simulink model "xo_test"  (R2023a)
settings: Solver=VariableStepAuto  StartTime=0.0  StopTime=10.0  RelTol=1e-3
PreLoadFcn:
  | xo = importrobot('urdf/alpha4_LC_FB_XYZ.urdf');
  | xo.DataFormat = 'col';
libraries: robotmaniplib x72, RoboticsCode x72
(part 2 of 2)

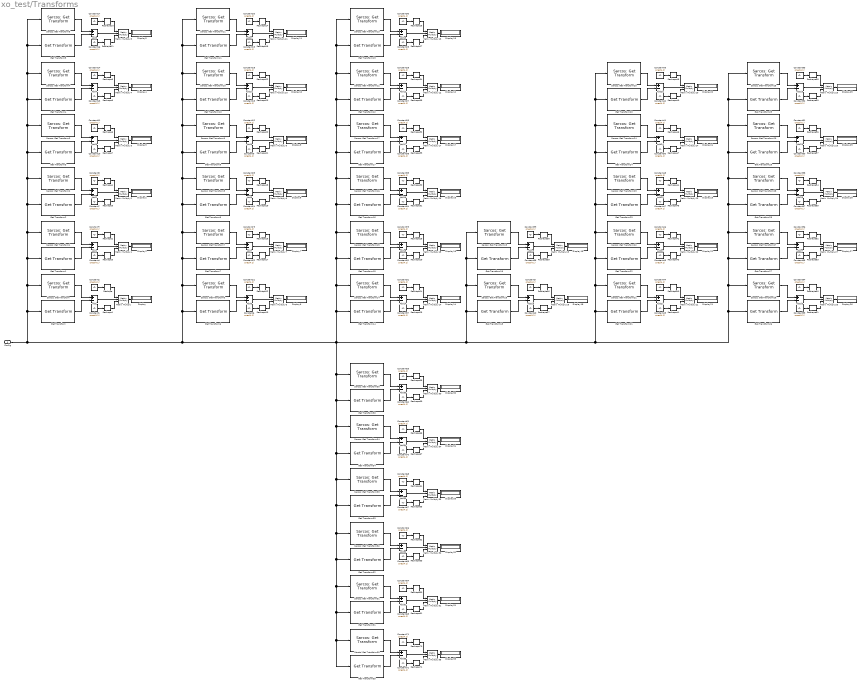
== system xo_test/Transforms ==
  Config : Inport
  Add{,1..35} (36 alike) : Sum  Inputs=+-
  Constant{1..72} (72 alike) : Constant  Value=ones(4,1)
  Display{,1..35} (36 alike) : Display
  Get Transform : robotmaniplib/Get Transform  RigidBodyTree=xo  SourceBody=BaseRotZ  TargetBody=World  SimulateUsing=Interpreted execution
  Get Transform1 : robotmaniplib/Get Transform  RigidBodyTree=xo  SourceBody=BaseRotY  TargetBody=World  SimulateUsing=Interpreted execution
  Get Transform10 : robotmaniplib/Get Transform  RigidBodyTree=xo  SourceBody=LeftHipAbAd  TargetBody=World  SimulateUsing=Interpreted execution
  Get Transform11 : robotmaniplib/Get Transform  RigidBodyTree=xo  SourceBody=LeftHipRotate  TargetBody=World  SimulateUsing=Interpreted execution
  Get Transform12 : robotmaniplib/Get Transform  RigidBodyTree=xo  SourceBody=BasePosY  TargetBody=World  SimulateUsing=Interpreted execution
  Get Transform13 : robotmaniplib/Get Transform  RigidBodyTree=xo  SourceBody=BasePosX  TargetBody=World  SimulateUsing=Interpreted execution
  Get Transform14 : robotmaniplib/Get Transform  RigidBodyTree=xo  SourceBody=BaseRotZ  TargetBody=World  SimulateUsing=Interpreted execution
  Get Transform15 : robotmaniplib/Get Transform  RigidBodyTree=xo  SourceBody=BaseRotY  TargetBody=World  SimulateUsing=Interpreted execution
  Get Transform16 : robotmaniplib/Get Transform  RigidBodyTree=xo  SourceBody=BaseRotX  TargetBody=World  SimulateUsing=Interpreted execution
  Get Transform17 : robotmaniplib/Get Transform  RigidBodyTree=xo  SourceBody=BasePosZ  TargetBody=World  SimulateUsing=Interpreted execution
  Get Transform18 : robotmaniplib/Get Transform  RigidBodyTree=xo  SourceBody=TorsoRotate  TargetBody=World  SimulateUsing=Interpreted execution
  Get Transform19 : robotmaniplib/Get Transform  RigidBodyTree=xo  SourceBody=TorsoTilt  TargetBody=World  SimulateUsing=Interpreted execution
  Get Transform2 : robotmaniplib/Get Transform  RigidBodyTree=xo  SourceBody=BaseRotX  TargetBody=World  SimulateUsing=Interpreted execution
  Get Transform20 : robotmaniplib/Get Transform  RigidBodyTree=xo  SourceBody=LeftShoulderAbAd  TargetBody=World  SimulateUsing=Interpreted execution
  Get Transform21 : robotmaniplib/Get Transform  RigidBodyTree=xo  SourceBody=LeftWristRotate  TargetBody=World  SimulateUsing=Interpreted execution
  Get Transform22 : robotmaniplib/Get Transform  RigidBodyTree=xo  SourceBody=LeftElbowFlex  TargetBody=World  SimulateUsing=Interpreted execution
  Get Transform23 : robotmaniplib/Get Transform  RigidBodyTree=xo  SourceBody=LeftHumeralRotate  TargetBody=World  SimulateUsing=Interpreted execution
  Get Transform24 : robotmaniplib/Get Transform  RigidBodyTree=xo  SourceBody=LeftShoulderFlex  TargetBody=World  SimulateUsing=Interpreted execution
  Get Transform25 : robotmaniplib/Get Transform  RigidBodyTree=xo  SourceBody=RightShoulderAbAd  TargetBody=World  SimulateUsing=Interpreted execution
  Get Transform26 : robotmaniplib/Get Transform  RigidBodyTree=xo  SourceBody=RightWristRotate  TargetBody=World  SimulateUsing=Interpreted execution
  Get Transform27 : robotmaniplib/Get Transform  RigidBodyTree=xo  SourceBody=RightElbowFlex  TargetBody=World  SimulateUsing=Interpreted execution
  Get Transform28 : robotmaniplib/Get Transform  RigidBodyTree=xo  SourceBody=RightHumeralRotate  TargetBody=World  SimulateUsing=Interpreted execution
  Get Transform29 : robotmaniplib/Get Transform  RigidBodyTree=xo  SourceBody=RightShoulderFlex  TargetBody=World  SimulateUsing=Interpreted execution
  Get Transform3 : robotmaniplib/Get Transform  RigidBodyTree=xo  SourceBody=BasePosZ  TargetBody=World  SimulateUsing=Interpreted execution
  Get Transform30 : robotmaniplib/Get Transform  RigidBodyTree=xo  SourceBody=PelvisLoadCell  TargetBody=World  SimulateUsing=Interpreted execution
  Get Transform31 : robotmaniplib/Get Transform  RigidBodyTree=xo  SourceBody=LeftHandleLoadCell  TargetBody=World  SimulateUsing=Interpreted execution
  Get Transform32 : robotmaniplib/Get Transform  RigidBodyTree=xo  SourceBody=TorsoLoadCell  TargetBody=World  SimulateUsing=Interpreted execution
  Get Transform33 : robotmaniplib/Get Transform  RigidBodyTree=xo  SourceBody=RightFootLoadCell  TargetBody=World  SimulateUsing=Interpreted execution
  Get Transform34 : robotmaniplib/Get Transform  RigidBodyTree=xo  SourceBody=LeftFootLoadCell  TargetBody=World  SimulateUsing=Interpreted execution
  Get Transform35 : robotmaniplib/Get Transform  RigidBodyTree=xo  SourceBody=RightHandleLoadCell  TargetBody=World  SimulateUsing=Interpreted execution
  Get Transform4 : robotmaniplib/Get Transform  RigidBodyTree=xo  SourceBody=BasePosY  TargetBody=World  SimulateUsing=Interpreted execution
  Get Transform5 : robotmaniplib/Get Transform  RigidBodyTree=xo  SourceBody=BasePosX  TargetBody=World  SimulateUsing=Interpreted execution
  Get Transform6 : robotmaniplib/Get Transform  RigidBodyTree=xo  SourceBody=LeftAnkleFlex  TargetBody=World  SimulateUsing=Interpreted execution
  Get Transform7 : robotmaniplib/Get Transform  RigidBodyTree=xo  SourceBody=LeftCalfRotate  TargetBody=World  SimulateUsing=Interpreted execution
  Get Transform8 : robotmaniplib/Get Transform  RigidBodyTree=xo  SourceBody=LeftKneeFlex  TargetBody=World  SimulateUsing=Interpreted execution
  Get Transform9 : robotmaniplib/Get Transform  RigidBodyTree=xo  SourceBody=LeftHipFlex  TargetBody=World  SimulateUsing=Interpreted execution
  Matrix Multiply{,1..35} (36 alike) : Product  Inputs=3  Multiplication=Matrix(*)
  Reshape{,2,4,6,8,10,12,14,16,18,20,22,24,26,28,30,32,34,36,38,40,42,44,46,48,50,52,54,56,58,60,62,64,66,68,70} (36 alike) : Reshape  OutputDimensionality=Row vector (2-D)
  Reshape{1,3,5,7,9,11,13,15,17,19,21,23,25,27,29,31,33,35,37,39,41,43,45,47,49,51,53,55,57,59,61,63,65,67,69,71} (36 alike) : Reshape  OutputDimensionality=Column vector (2-D)
  Sarcos: Get Transform : RoboticsCode/Sarcos: Get Transform  urdfpath='alpha4_LC_FB_XYZ.urdf'  source=BaseRotZ  source_string='BaseRotZ'  target=World  target_string='World'
      settings: SourceProductName=Sacros Robotics Toolbox
  Sarcos: Get Transform1 : RoboticsCode/Sarcos: Get Transform  urdfpath='alpha4_LC_FB_XYZ.urdf'  source=BaseRotY  source_string='BaseRotY'  target=World  target_string='World'
      settings: SourceProductName=Sacros Robotics Toolbox
  Sarcos: Get Transform10 : RoboticsCode/Sarcos: Get Transform  urdfpath='alpha4_LC_FB_XYZ.urdf'  source=LeftHipAbAd  source_string='LeftHipAbAd'  target=World  target_string='World'
      settings: SourceProductName=Sacros Robotics Toolbox
  Sarcos: Get Transform11 : RoboticsCode/Sarcos: Get Transform  urdfpath='alpha4_LC_FB_XYZ.urdf'  source=LeftHipRotate  source_string='LeftHipRotate'  target=World  target_string='World'
      settings: SourceProductName=Sacros Robotics Toolbox
  Sarcos: Get Transform12 : RoboticsCode/Sarcos: Get Transform  urdfpath='alpha4_LC_FB_XYZ.urdf'  source=BasePosY  source_string='BasePosY'  target=World  target_string='World'
      settings: SourceProductName=Sacros Robotics Toolbox
  Sarcos: Get Transform13 : RoboticsCode/Sarcos: Get Transform  urdfpath='alpha4_LC_FB_XYZ.urdf'  source=BasePosX  source_string='BasePosX'  target=World  target_string='World'
      settings: SourceProductName=Sacros Robotics Toolbox
  Sarcos: Get Transform14 : RoboticsCode/Sarcos: Get Transform  urdfpath='alpha4_LC_FB_XYZ.urdf'  source=BaseRotZ  source_string='BaseRotZ'  target=World  target_string='World'
      settings: SourceProductName=Sacros Robotics Toolbox
  Sarcos: Get Transform15 : RoboticsCode/Sarcos: Get Transform  urdfpath='alpha4_LC_FB_XYZ.urdf'  source=BaseRotY  source_string='BaseRotY'  target=World  target_string='World'
      settings: SourceProductName=Sacros Robotics Toolbox
  Sarcos: Get Transform16 : RoboticsCode/Sarcos: Get Transform  urdfpath='alpha4_LC_FB_XYZ.urdf'  source=BaseRotX  source_string='BaseRotX'  target=World  target_string='World'
      settings: SourceProductName=Sacros Robotics Toolbox
  Sarcos: Get Transform17 : RoboticsCode/Sarcos: Get Transform  urdfpath='alpha4_LC_FB_XYZ.urdf'  source=BasePosZ  source_string='BasePosZ'  target=World  target_string='World'
      settings: SourceProductName=Sacros Robotics Toolbox
  Sarcos: Get Transform18 : RoboticsCode/Sarcos: Get Transform  urdfpath='alpha4_LC_FB_XYZ.urdf'  source=TorsoRotate  source_string='TorsoRotate'  target=World  target_string='World'
      settings: SourceProductName=Sacros Robotics Toolbox
  Sarcos: Get Transform19 : RoboticsCode/Sarcos: Get Transform  urdfpath='alpha4_LC_FB_XYZ.urdf'  source=TorsoTilt  source_string='TorsoTilt'  target=World  target_string='World'
      settings: SourceProductName=Sacros Robotics Toolbox
  Sarcos: Get Transform2 : RoboticsCode/Sarcos: Get Transform  urdfpath='alpha4_LC_FB_XYZ.urdf'  source=BaseRotX  source_string='BaseRotX'  target=World  target_string='World'
      settings: SourceProductName=Sacros Robotics Toolbox
  Sarcos: Get Transform20 : RoboticsCode/Sarcos: Get Transform  urdfpath='alpha4_LC_FB_XYZ.urdf'  source=LeftShoulderAbAd  source_string='LeftShoulderAbAd'  target=World  target_string='World'
      settings: SourceProductName=Sacros Robotics Toolbox
  Sarcos: Get Transform21 : RoboticsCode/Sarcos: Get Transform  urdfpath='alpha4_LC_FB_XYZ.urdf'  source=LeftWristRotate  source_string='LeftWristRotate'  target=World  target_string='World'
      settings: SourceProductName=Sacros Robotics Toolbox
  Sarcos: Get Transform22 : RoboticsCode/Sarcos: Get Transform  urdfpath='alpha4_LC_FB_XYZ.urdf'  source=LeftElbowFlex  source_string='LeftElbowFlex'  target=World  target_string='World'
      settings: SourceProductName=Sacros Robotics Toolbox
  Sarcos: Get Transform23 : RoboticsCode/Sarcos: Get Transform  urdfpath='alpha4_LC_FB_XYZ.urdf'  source=LeftHumeralRotate  source_string='LeftHumeralRotate'  target=World  target_string='World'
      settings: SourceProductName=Sacros Robotics Toolbox
  Sarcos: Get Transform24 : RoboticsCode/Sarcos: Get Transform  urdfpath='alpha4_LC_FB_XYZ.urdf'  source=LeftShoulderFlex  source_string='LeftShoulderFlex'  target=World  target_string='World'
      settings: SourceProductName=Sacros Robotics Toolbox
  Sarcos: Get Transform25 : RoboticsCode/Sarcos: Get Transform  urdfpath='alpha4_LC_FB_XYZ.urdf'  source=RightShoulderAbAd  source_string='RightShoulderAbAd'  target=World  target_string='World'
      settings: SourceProductName=Sacros Robotics Toolbox
  Sarcos: Get Transform26 : RoboticsCode/Sarcos: Get Transform  urdfpath='alpha4_LC_FB_XYZ.urdf'  source=RightWristRotate  source_string='RightWristRotate'  target=World  target_string='World'
      settings: SourceProductName=Sacros Robotics Toolbox
  Sarcos: Get Transform27 : RoboticsCode/Sarcos: Get Transform  urdfpath='alpha4_LC_FB_XYZ.urdf'  source=RightElbowFlex  source_string='RightElbowFlex'  target=World  target_string='World'
      settings: SourceProductName=Sacros Robotics Toolbox
  Sarcos: Get Transform28 : RoboticsCode/Sarcos: Get Transform  urdfpath='alpha4_LC_FB_XYZ.urdf'  source=RightHumeralRotate  source_string='RightHumeralRotate'  target=World  target_string='World'
      settings: SourceProductName=Sacros Robotics Toolbox
  Sarcos: Get Transform29 : RoboticsCode/Sarcos: Get Transform  urdfpath='alpha4_LC_FB_XYZ.urdf'  source=RightShoulderFlex  source_string='RightShoulderFlex'  target=World  target_string='World'
      settings: SourceProductName=Sacros Robotics Toolbox
  Sarcos: Get Transform3 : RoboticsCode/Sarcos: Get Transform  urdfpath='alpha4_LC_FB_XYZ.urdf'  source=BasePosZ  source_string='BasePosZ'  target=World  target_string='World'
      settings: SourceProductName=Sacros Robotics Toolbox
  Sarcos: Get Transform30 : RoboticsCode/Sarcos: Get Transform  urdfpath='alpha4_LC_FB_XYZ.urdf'  source=PelvisLoadCell  source_string='PelvisLoadCell'  target=World  target_string='World'
      settings: SourceProductName=Sacros Robotics Toolbox
  Sarcos: Get Transform31 : RoboticsCode/Sarcos: Get Transform  urdfpath='alpha4_LC_FB_XYZ.urdf'  source=LeftHandleLoadCell  source_string='LeftHandleLoadCell'  target=World  target_string='World'
      settings: SourceProductName=Sacros Robotics Toolbox
  Sarcos: Get Transform32 : RoboticsCode/Sarcos: Get Transform  urdfpath='alpha4_LC_FB_XYZ.urdf'  source=TorsoLoadCell  source_string='TorsoLoadCell'  target=World  target_string='World'
      settings: SourceProductName=Sacros Robotics Toolbox
  Sarcos: Get Transform33 : RoboticsCode/Sarcos: Get Transform  urdfpath='alpha4_LC_FB_XYZ.urdf'  source=RightFootLoadCell  source_string='RightFootLoadCell'  target=World  target_string='World'
      settings: SourceProductName=Sacros Robotics Toolbox
  Sarcos: Get Transform34 : RoboticsCode/Sarcos: Get Transform  urdfpath='alpha4_LC_FB_XYZ.urdf'  source=LeftFootLoadCell  source_string='LeftFootLoadCell'  target=World  target_string='World'
      settings: SourceProductName=Sacros Robotics Toolbox
  Sarcos: Get Transform35 : RoboticsCode/Sarcos: Get Transform  urdfpath='alpha4_LC_FB_XYZ.urdf'  source=RightHandleLoadCell  source_string='RightHandleLoadCell'  target=World  target_string='World'
      settings: SourceProductName=Sacros Robotics Toolbox
  Sarcos: Get Transform4 : RoboticsCode/Sarcos: Get Transform  urdfpath='alpha4_LC_FB_XYZ.urdf'  source=BasePosY  source_string='BasePosY'  target=World  target_string='World'
      settings: SourceProductName=Sacros Robotics Toolbox
  Sarcos: Get Transform5 : RoboticsCode/Sarcos: Get Transform  urdfpath='alpha4_LC_FB_XYZ.urdf'  source=BasePosX  source_string='BasePosX'  target=World  target_string='World'
      settings: SourceProductName=Sacros Robotics Toolbox
  Sarcos: Get Transform6 : RoboticsCode/Sarcos: Get Transform  urdfpath='alpha4_LC_FB_XYZ.urdf'  source=LeftAnkleFlex  source_string='LeftAnkleFlex'  target=World  target_string='World'
      settings: SourceProductName=Sacros Robotics Toolbox
  Sarcos: Get Transform7 : RoboticsCode/Sarcos: Get Transform  urdfpath='alpha4_LC_FB_XYZ.urdf'  source=LeftCalfRotate  source_string='LeftCalfRotate'  target=World  target_string='World'
      settings: SourceProductName=Sacros Robotics Toolbox
  Sarcos: Get Transform8 : RoboticsCode/Sarcos: Get Transform  urdfpath='alpha4_LC_FB_XYZ.urdf'  source=LeftKneeFlex  source_string='LeftKneeFlex'  target=World  target_string='World'
      settings: SourceProductName=Sacros Robotics Toolbox
  Sarcos: Get Transform9 : RoboticsCode/Sarcos: Get Transform  urdfpath='alpha4_LC_FB_XYZ.urdf'  source=LeftHipFlex  source_string='LeftHipFlex'  target=World  target_string='World'
      settings: SourceProductName=Sacros Robotics Toolbox
  wires:
  Config/1 -> Get Transform2/1, Sarcos: Get Transform5/1, Get Transform5/1, Sarcos: Get Transform4/1, Get Transform4/1, Sarcos: Get Transform3/1, Get Transform3/1, Sarcos: Get Transform2/1, Sarcos: Get Transform1/1, Get Transform1/1, Sarcos: Get Transform/1, Get Transform/1, Get Transform33/1, Sarcos: Get Transform32/1, Sarcos: Get Transform31/1, Get Transform35/1, Sarcos: Get Transform35/1, Get Transform31/1, Get Transform32/1, Sarcos: Get Transform33/1, Get Transform34/1, Sarcos: Get Transform34/1, Get Transform30/1, Sarcos: Get Transform30/1, Get Transform16/1, Sarcos: Get Transform13/1, Get Transform13/1, Sarcos: Get Transform12/1, Get Transform12/1, Sarcos: Get Transform17/1, Get Transform17/1, Sarcos: Get Transform16/1, Sarcos: Get Transform15/1, Get Transform15/1, Sarcos: Get Transform14/1, Get Transform14/1, Sarcos: Get Transform25/1, Get Transform25/1, Sarcos: Get Transform29/1, Get Transform29/1, Sarcos: Get Transform28/1, Get Transform28/1, Sarcos: Get Transform27/1, Get Transform27/1, Sarcos: Get Transform26/1, Get Transform26/1, Get Transform24/1, Sarcos: Get Transform20/1, Get Transform20/1, Sarcos: Get Transform24/1, Sarcos: Get Transform23/1, Get Transform23/1, Sarcos: Get Transform22/1, Get Transform22/1, Sarcos: Get Transform21/1, Get Transform21/1, Sarcos: Get Transform19/1, Get Transform19/1, Sarcos: Get Transform18/1, Get Transform18/1, Sarcos: Get Transform6/1, Get Transform7/1, Sarcos: Get Transform7/1, Sarcos: Get Transform8/1, Get Transform9/1, Sarcos: Get Transform9/1, Get Transform10/1, Sarcos: Get Transform10/1, Get Transform11/1, Sarcos: Get Transform11/1, Get Transform8/1, Get Transform6/1
  Matrix Multiply4/1 -> Display4/1
  Reshape33/1 -> Matrix Multiply17/3
  Sarcos: Get Transform17/1 -> Add17/1
  Add1/1 -> Matrix Multiply1/2
  Reshape10/1 -> Matrix Multiply5/1
  Get Transform13/1 -> Add13/2
  Get Transform10/1 -> Add10/2
  Sarcos: Get Transform10/1 -> Add10/1
  Reshape35/1 -> Matrix Multiply12/3
  Add13/1 -> Matrix Multiply13/2
  Constant33/1 -> Reshape28/1
  Matrix Multiply8/1 -> Display8/1
  Add17/1 -> Matrix Multiply17/2
  Constant7/1 -> Reshape5/1
  Reshape3/1 -> Matrix Multiply1/3
  Constant26/1 -> Reshape32/1
  Reshape32/1 -> Matrix Multiply17/1
  Sarcos: Get Transform14/1 -> Add14/1
  Constant24/1 -> Reshape19/1
  Reshape4/1 -> Matrix Multiply2/1
  Sarcos: Get Transform11/1 -> Add11/1
  Get Transform17/1 -> Add17/2
  Reshape28/1 -> Matrix Multiply15/1
  Constant35/1 -> Reshape30/1
  Constant10/1 -> Reshape7/1
  Reshape9/1 -> Matrix Multiply4/3
  Reshape18/1 -> Matrix Multiply8/1
  Constant27/1 -> Reshape35/1
  Matrix Multiply10/1 -> Display10/1
  Constant8/1 -> Reshape4/1
  Reshape5/1 -> Matrix Multiply2/3
  Matrix Multiply16/1 -> Display16/1
  Add15/1 -> Matrix Multiply15/2
  Reshape34/1 -> Matrix Multiply12/1
  Matrix Multiply17/1 -> Display17/1
  Constant38/1 -> Reshape33/1
  Constant29/1 -> Reshape27/1
  Reshape29/1 -> Matrix Multiply15/3
  Reshape31/1 -> Matrix Multiply16/3
  Sarcos: Get Transform2/1 -> Add2/1
  Reshape19/1 -> Matrix Multiply8/3
  Matrix Multiply13/1 -> Display13/1
  Get Transform14/1 -> Add14/2
  Sarcos: Get Transform16/1 -> Add16/1
  Constant4/1 -> Reshape3/1
  Sarcos: Get Transform/1 -> Add/1
  Get Transform16/1 -> Add16/2
  Reshape24/1 -> Matrix Multiply14/1
  Reshape17/1 -> Matrix Multiply7/3
  Sarcos: Get Transform12/1 -> Add12/1
  Sarcos: Get Transform15/1 -> Add15/1
  Reshape30/1 -> Matrix Multiply16/1
  Matrix Multiply3/1 -> Display3/1
  Constant21/1 -> Reshape12/1
  Matrix Multiply14/1 -> Display14/1
  Constant37/1 -> Reshape25/1
  Add16/1 -> Matrix Multiply16/2
  Constant17/1 -> Reshape10/1
  Constant16/1 -> Reshape11/1
  Constant31/1 -> Reshape24/1
  Constant34/1 -> Reshape31/1
  Add14/1 -> Matrix Multiply14/2
  Constant32/1 -> Reshape29/1
  Get Transform15/1 -> Add15/2
  Add12/1 -> Matrix Multiply12/2
  Reshape25/1 -> Matrix Multiply14/3
  Matrix Multiply15/1 -> Display15/1
  Reshape26/1 -> Matrix Multiply13/1
  Reshape27/1 -> Matrix Multiply13/3
  Add7/1 -> Matrix Multiply7/2
  Constant30/1 -> Reshape26/1
  Get Transform12/1 -> Add12/2
  Sarcos: Get Transform13/1 -> Add13/1
  Matrix Multiply12/1 -> Display12/1
  Get Transform7/1 -> Add7/2
  Constant28/1 -> Reshape34/1
  Constant23/1 -> Reshape16/1
  Constant5/1 -> Reshape2/1
  Reshape20/1 -> Matrix Multiply9/1
  Add/1 -> Matrix Multiply/2
  Matrix Multiply7/1 -> Display7/1
  Constant22/1 -> Reshape17/1
  Reshape16/1 -> Matrix Multiply7/1
  Reshape12/1 -> Matrix Multiply6/1
  Constant20/1 -> Reshape14/1
  Matrix Multiply5/1 -> Display5/1
  Reshape13/1 -> Matrix Multiply6/3
  Constant6/1 -> Reshape13/1
  Matrix Multiply6/1 -> Display6/1
  Add6/1 -> Matrix Multiply6/2
  Sarcos: Get Transform6/1 -> Add6/1
  Get Transform6/1 -> Add6/2
  Add8/1 -> Matrix Multiply8/2
  Constant18/1 -> Reshape22/1
  Sarcos: Get Transform9/1 -> Add9/1
  Add9/1 -> Matrix Multiply9/2
  Get Transform9/1 -> Add9/2
  Matrix Multiply9/1 -> Display9/1
  Constant9/1 -> Reshape21/1
  Constant12/1 -> Reshape20/1
  Reshape21/1 -> Matrix Multiply9/3
  Reshape22/1 -> Matrix Multiply10/1
  Reshape23/1 -> Matrix Multiply10/3
  Constant19/1 -> Reshape15/1
  Constant15/1 -> Reshape23/1
  Add11/1 -> Matrix Multiply11/2
  Matrix Multiply11/1 -> Display11/1
  Get Transform11/1 -> Add11/2
  Add10/1 -> Matrix Multiply10/2
  Reshape14/1 -> Matrix Multiply11/1
  Constant25/1 -> Reshape18/1
  Reshape15/1 -> Matrix Multiply11/3
  Sarcos: Get Transform3/1 -> Add3/1
  Sarcos: Get Transform7/1 -> Add7/1
  Get Transform8/1 -> Add8/2
  Sarcos: Get Transform8/1 -> Add8/1
  Get Transform/1 -> Add/2
  Reshape11/1 -> Matrix Multiply5/3
  Get Transform5/1 -> Add5/2
  Sarcos: Get Transform5/1 -> Add5/1
  Add5/1 -> Matrix Multiply5/2
  Get Transform4/1 -> Add4/2
  Sarcos: Get Transform4/1 -> Add4/1
  Constant14/1 -> Reshape8/1
  Constant1/1 -> Reshape1/1
  Add4/1 -> Matrix Multiply4/2
  Constant13/1 -> Reshape9/1
  Reshape7/1 -> Matrix Multiply3/3
  Reshape6/1 -> Matrix Multiply3/1
  Reshape8/1 -> Matrix Multiply4/1
  Constant11/1 -> Reshape6/1
  Add3/1 -> Matrix Multiply3/2
  Get Transform3/1 -> Add3/2
  Constant2/1 -> Reshape/1
  Get Transform1/1 -> Add1/2
  Sarcos: Get Transform1/1 -> Add1/1
  Add2/1 -> Matrix Multiply2/2
  Reshape2/1 -> Matrix Multiply1/1
  Matrix Multiply1/1 -> Display1/1
  Reshape/1 -> Matrix Multiply/1
  Get Transform2/1 -> Add2/2
  Matrix Multiply2/1 -> Display2/1
  Matrix Multiply/1 -> Display/1
  Reshape1/1 -> Matrix Multiply/3
  Matrix Multiply19/1 -> Display19/1
  Reshape37/1 -> Matrix Multiply18/3
  Get Transform19/1 -> Add19/2
  Constant36/1 -> Reshape39/1
  Add18/1 -> Matrix Multiply18/2
  Constant3/1 -> Reshape36/1
  Constant40/1 -> Reshape37/1
  Matrix Multiply18/1 -> Display18/1
  Sarcos: Get Transform19/1 -> Add19/1
  Reshape36/1 -> Matrix Multiply18/1
  Get Transform18/1 -> Add18/2
  Reshape39/1 -> Matrix Multiply19/3
  Add19/1 -> Matrix Multiply19/2
  Reshape38/1 -> Matrix Multiply19/1
  Sarcos: Get Transform18/1 -> Add18/1
  Constant39/1 -> Reshape38/1
  Constant43/1 -> Reshape48/1
  Matrix Multiply20/1 -> Display20/1
  Get Transform20/1 -> Add20/2
  Matrix Multiply22/1 -> Display22/1
  Reshape41/1 -> Matrix Multiply21/3
  Add20/1 -> Matrix Multiply20/2
  Get Transform22/1 -> Add22/2
  Constant45/1 -> Reshape43/1
  Add21/1 -> Matrix Multiply21/2
  Constant47/1 -> Reshape45/1
  Constant44/1 -> Reshape40/1
  Add23/1 -> Matrix Multiply23/2
  Constant49/1 -> Reshape41/1
  Matrix Multiply21/1 -> Display21/1
  Reshape44/1 -> Matrix Multiply23/1
  Sarcos: Get Transform22/1 -> Add22/1
  Sarcos: Get Transform20/1 -> Add20/1
  Reshape40/1 -> Matrix Multiply21/1
  Get Transform23/1 -> Add23/2
  Sarcos: Get Transform23/1 -> Add23/1
  Get Transform21/1 -> Add21/2
  Reshape45/1 -> Matrix Multiply23/3
  Reshape43/1 -> Matrix Multiply22/3
  Constant50/1 -> Reshape47/1
  Matrix Multiply24/1 -> Display24/1
  Reshape48/1 -> Matrix Multiply20/1
  Add22/1 -> Matrix Multiply22/2
  Matrix Multiply23/1 -> Display23/1
  Constant42/1 -> Reshape49/1
  Constant48/1 -> Reshape44/1
  Reshape42/1 -> Matrix Multiply22/1
  Get Transform24/1 -> Add24/2
  Sarcos: Get Transform21/1 -> Add21/1
  Reshape46/1 -> Matrix Multiply24/1
  Constant41/1 -> Reshape46/1
  Add24/1 -> Matrix Multiply24/2
  Constant46/1 -> Reshape42/1
  Reshape49/1 -> Matrix Multiply20/3
  Sarcos: Get Transform24/1 -> Add24/1
  Reshape47/1 -> Matrix Multiply24/3
  Reshape57/1 -> Matrix Multiply29/3
  Sarcos: Get Transform29/1 -> Add29/1
  Reshape59/1 -> Matrix Multiply25/3
  Constant56/1 -> Reshape52/1
  Add29/1 -> Matrix Multiply29/2
  Constant51/1 -> Reshape56/1
  Reshape56/1 -> Matrix Multiply29/1
  Sarcos: Get Transform26/1 -> Add26/1
  Get Transform29/1 -> Add29/2
  Reshape52/1 -> Matrix Multiply27/1
  Constant58/1 -> Reshape54/1
  Constant52/1 -> Reshape59/1
  Matrix Multiply28/1 -> Display28/1
  Add27/1 -> Matrix Multiply27/2
  Reshape58/1 -> Matrix Multiply25/1
  Matrix Multiply29/1 -> Display29/1
  Constant60/1 -> Reshape57/1
  Reshape53/1 -> Matrix Multiply27/3
  Reshape55/1 -> Matrix Multiply28/3
  Get Transform26/1 -> Add26/2
  Sarcos: Get Transform28/1 -> Add28/1
  Get Transform28/1 -> Add28/2
  Reshape50/1 -> Matrix Multiply26/1
  Sarcos: Get Transform25/1 -> Add25/1
  Sarcos: Get Transform27/1 -> Add27/1
  Reshape54/1 -> Matrix Multiply28/1
  Matrix Multiply26/1 -> Display26/1
  Constant59/1 -> Reshape51/1
  Add28/1 -> Matrix Multiply28/2
  Constant54/1 -> Reshape50/1
  Constant57/1 -> Reshape55/1
  Add26/1 -> Matrix Multiply26/2
  Constant55/1 -> Reshape53/1
  Get Transform27/1 -> Add27/2
  Add25/1 -> Matrix Multiply25/2
  Reshape51/1 -> Matrix Multiply26/3
  Matrix Multiply27/1 -> Display27/1
  Get Transform25/1 -> Add25/2
  Matrix Multiply25/1 -> Display25/1
  Constant53/1 -> Reshape58/1
  Constant63/1 -> Reshape68/1
  Matrix Multiply30/1 -> Display30/1
  Get Transform30/1 -> Add30/2
  Matrix Multiply32/1 -> Display32/1
  Reshape61/1 -> Matrix Multiply31/3
  Add30/1 -> Matrix Multiply30/2
  Get Transform32/1 -> Add32/2
  Constant65/1 -> Reshape63/1
  Add31/1 -> Matrix Multiply31/2
  Constant67/1 -> Reshape65/1
  Constant64/1 -> Reshape60/1
  Add33/1 -> Matrix Multiply33/2
  Constant69/1 -> Reshape61/1
  Matrix Multiply31/1 -> Display31/1
  Reshape64/1 -> Matrix Multiply33/1
  Sarcos: Get Transform32/1 -> Add32/1
  Sarcos: Get Transform30/1 -> Add30/1
  Reshape60/1 -> Matrix Multiply31/1
  Get Transform33/1 -> Add33/2
  Sarcos: Get Transform33/1 -> Add33/1
  Get Transform31/1 -> Add31/2
  Reshape65/1 -> Matrix Multiply33/3
  Reshape63/1 -> Matrix Multiply32/3
  Constant70/1 -> Reshape67/1
  Matrix Multiply34/1 -> Display34/1
  Reshape68/1 -> Matrix Multiply30/1
  Add32/1 -> Matrix Multiply32/2
  Matrix Multiply33/1 -> Display33/1
  Constant62/1 -> Reshape69/1
  Constant68/1 -> Reshape64/1
  Reshape62/1 -> Matrix Multiply32/1
  Get Transform34/1 -> Add34/2
  Sarcos: Get Transform31/1 -> Add31/1
  Reshape66/1 -> Matrix Multiply34/1
  Constant61/1 -> Reshape66/1
  Add34/1 -> Matrix Multiply34/2
  Constant66/1 -> Reshape62/1
  Reshape69/1 -> Matrix Multiply30/3
  Sarcos: Get Transform34/1 -> Add34/1
  Reshape67/1 -> Matrix Multiply34/3
  Sarcos: Get Transform35/1 -> Add35/1
  Get Transform35/1 -> Add35/2
  Reshape70/1 -> Matrix Multiply35/1
  Matrix Multiply35/1 -> Display35/1
  Constant72/1 -> Reshape71/1
  Constant71/1 -> Reshape70/1
  Add35/1 -> Matrix Multiply35/2
  Reshape71/1 -> Matrix Multiply35/3
